simulink model "prob3"  (R2020b)
settings: Solver=VariableStepAuto  StartTime=0.0  StopTime=10.0  RelTol=1e-3
undefined symbols (not defined in the file): k1, k2
settings Model: Creator=Admin  LastModifiedBy=Admin

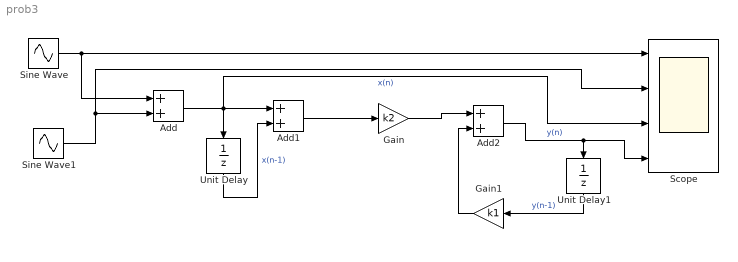
== system prob3 ==
  Add : Sum
  Add1 : Sum
  Add2 : Sum
  Gain : Gain  Gain=k2
  Gain1 : Gain  Gain=k1
  Scope : Scope  NumInputPorts=4
  Sine Wave : Sin  SampleTime=0
  Sine Wave1 : Sin  Frequency=50  SampleTime=0
  Unit Delay : UnitDelay  SampleTime=-1  HasFrameUpgradeWarning=on
  Unit Delay1 : UnitDelay  SampleTime=-1  HasFrameUpgradeWarning=on
  wires:
  Sine Wave/1 -> Add/1, Scope/1
  Sine Wave1/1 -> Add/2, Scope/2
  Add/1 -> Unit Delay/1, Scope/3, Add1/1  "x(n)"
  Unit Delay/1 -> Add1/2  "x(n-1)"
  Add1/1 -> Gain/1
  Gain/1 -> Add2/1
  Gain1/1 -> Add2/2
  Unit Delay1/1 -> Gain1/1  "y(n-1)"
  Add2/1 -> Unit Delay1/1, Scope/4  "y(n)"
